simulink model "SCCS_MIL_TestHarness_06"  (R2024a)
settings: Solver=ode3  StartTime=0.0  StopTime=10.0  FixedStep=0.01  RelTol=1e-3
settings Model: Creator=Kishore  LastModifiedBy=Kishore

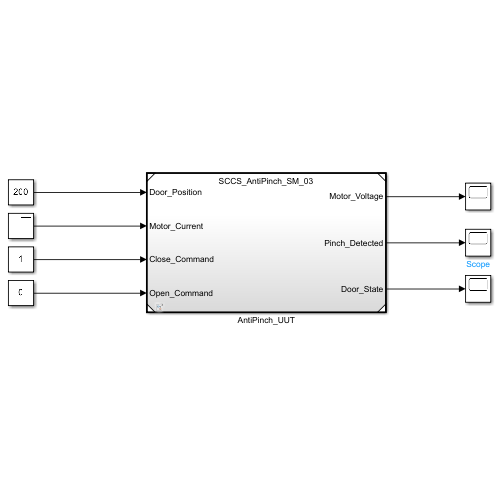
[thumbnail: Simulink's stored preview of the top-level diagram]
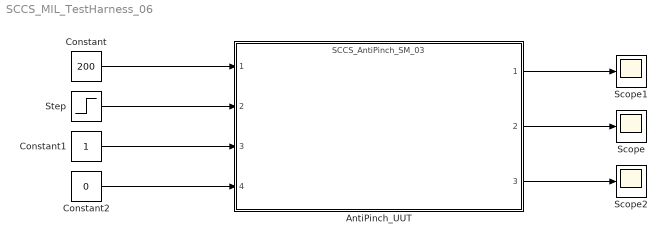
== system SCCS_MIL_TestHarness_06 ==
  AntiPinch_UUT : ModelReference  ModelNameDialog=SCCS_AntiPinch_SM_03.slx  SimulationMode=Normal  ModelReferenceVersion=1.13
  Constant : Constant  Value=200
  Constant1 : Constant
  Constant2 : Constant  Value=0
  Scope : Scope
  Scope1 : Scope
  Scope2 : Scope
  Step : Step  Time=2  Before=3  After=10  SampleTime=0
  wires:
  Constant/1 -> AntiPinch_UUT/1
  Constant1/1 -> AntiPinch_UUT/3
  Constant2/1 -> AntiPinch_UUT/4
  Step/1 -> AntiPinch_UUT/2
  AntiPinch_UUT/1 -> Scope1/1
  AntiPinch_UUT/2 -> Scope/1
  AntiPinch_UUT/3 -> Scope2/1
